simulink model "velocity"  (R2023b)
settings: Solver=VariableStepAuto  StartTime=0.0  StopTime=1  RelTol=1e-3
undefined symbols (not defined in the file): K, Ki
settings Model: Creator=Beniamino  LastModifiedBy=Beniamino

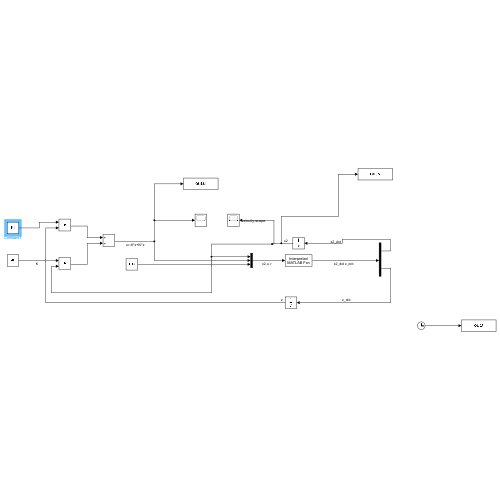
[thumbnail: Simulink's stored preview of the top-level diagram]
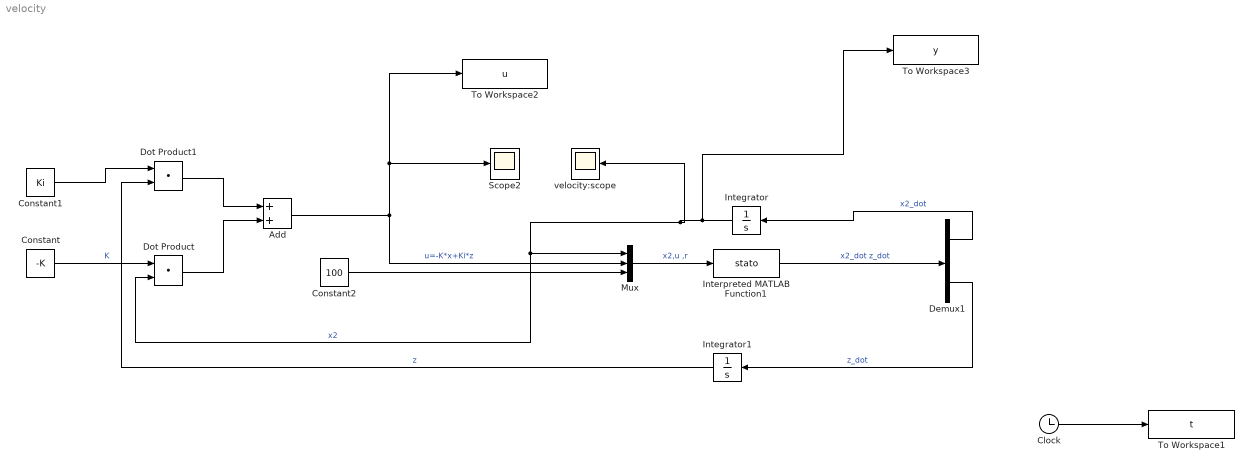
== system velocity ==
  Add : Sum
  Clock : Clock
  Constant : Constant  Value=-K
  Constant1 : Constant  Value=Ki
  Constant2 : Constant  Value=100
  Demux1 : Demux  Outputs=2
  Dot Product : DotProduct  OutDataTypeStr=Inherit: Inherit via internal rule
  Dot Product1 : DotProduct  OutDataTypeStr=Inherit: Inherit via internal rule
  Integrator : Integrator
  Integrator1 : Integrator
  Interpreted MATLAB Function1 : MATLABFcn  MATLABFcn=stato  OutputDimensions=2  Output1D=off
  Mux : Mux  Inputs=3
  Scope2 : Scope
  To Workspace1 : ToWorkspace  VariableName=t  SampleTime=-1
  To Workspace2 : ToWorkspace  VariableName=u  SampleTime=-1
  To Workspace3 : ToWorkspace  VariableName=y  SampleTime=-1
  velocity:scope : Scope
  wires:
  Constant/1 -> Dot Product/1  "K"
  Integrator/1 -> Mux/1, Dot Product/2, velocity:scope/1, To Workspace3/1  "x2"
  Dot Product/1 -> Add/2
  Constant1/1 -> Dot Product1/1
  Integrator1/1 -> Dot Product1/2  "z"
  Constant2/1 -> Mux/3
  Mux/1 -> Interpreted MATLAB Function1/1  "x2,u ,r"
  Interpreted MATLAB Function1/1 -> Demux1/1  "x2_dot z_dot"
  Demux1/2 -> Integrator1/1  "z_dot"
  Clock/1 -> To Workspace1/1
  Add/1 -> Mux/2, To Workspace2/1, Scope2/1  "u=-K*x+Ki*z"
  Demux1/1 -> Integrator/1  "x2_dot"
  Dot Product1/1 -> Add/1
